simulink model "walker"  (R2021a)
settings: Solver=ode15s  StartTime=0.0  StopTime=total_time  RelTol=1e-3
values from neighbouring files (symbols this model uses):
  I_trunk_xx = trunk.mass/20 * (trunk.depth^2 + trunk.height^2)    [createWalkerWithFixedStanceFootModel.m]
  I_trunk_yy = trunk.mass/20 * (trunk.width^2 + trunk.height^2)    [createWalkerWithFixedStanceFootModel.m]
  I_trunk_zz = trunk.mass/20 * (trunk.depth^2 + trunk.width^2)    [createWalkerWithFixedStanceFootModel.m]
  shank_com_from_ankle = geometry.ankle_to_knee_z / 2    [setBiomechanicsParameters.m]
  shank_com_from_knee = geometry.ankle_to_knee_z / 2    [setBiomechanicsParameters.m]
  tau = inverseDynamics(model, theta_init, theta_dot_init)    [initialize.m]
  theta_dot_init = [0; 0; 0; 0; 0; 0]    [initialize.m]
  theta_init = [IC.left_ankle_angle; IC.left_knee_angle; IC.left_hip_angle; IC.right_hip_angle; IC.right_knee_angle; IC.right_ankle_angle]    [initialize.m]
  thigh_com_from_hip = geometry.knee_to_hip_z / 2    [setBiomechanicsParameters.m]
  thigh_com_from_knee = geometry.knee_to_hip_z / 2    [setBiomechanicsParameters.m]
undefined symbols (not defined in the file or in its folder): foot, geometry, ground, head, shank, thigh, trunk, X, Y, Z
libraries: sm_lib x75, nesl_utility x26, Contact_Forces_Lib x8, Parts_Lib x8
(part 1 of 3)
settings Model: Creator=reimajbi  LastModifiedBy=reimajbi

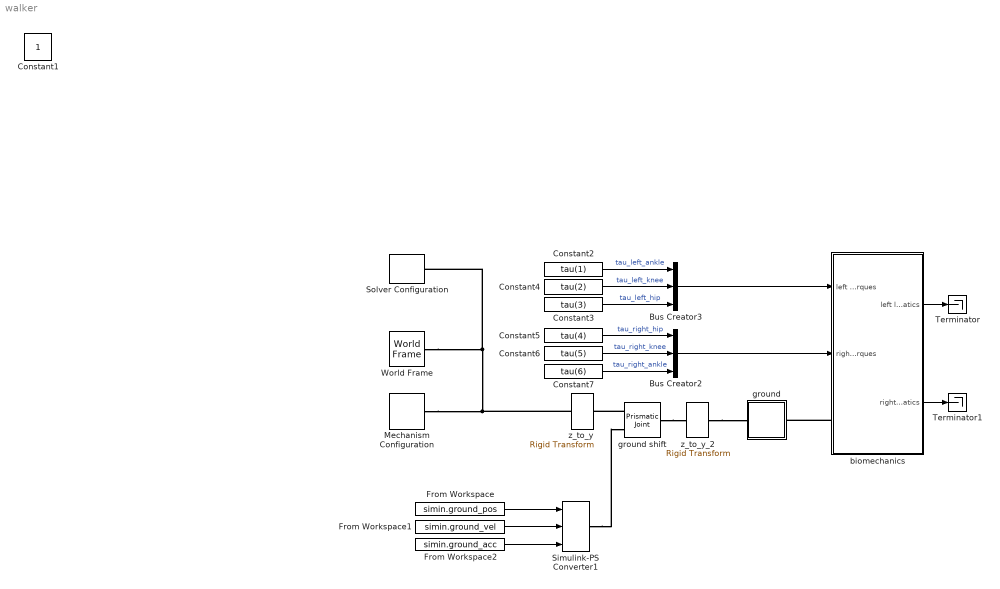
== system walker ==
  Bus Creator2 : BusCreator  Inputs=3
  Bus Creator3 : BusCreator  Inputs=3
  Constant2 : Constant  Value=tau(1)
  Constant3 : Constant  Value=tau(3)
  Constant4 : Constant  Value=tau(2)
  Constant5 : Constant  Value=tau(4)
  Constant6 : Constant  Value=tau(5)
  Constant7 : Constant  Value=tau(6)
  From Workspace : FromWorkspace  VariableName=simin.ground_pos
  From Workspace1 : FromWorkspace  VariableName=simin.ground_vel
  From Workspace2 : FromWorkspace  VariableName=simin.ground_acc
  Mechanism Configuration : sm_lib/Utilities/Mechanism Configuration  UniformGravity=Constant  GravityVector=[0 0 -9.80665]  GravityVectorUnits=m/s^2  GravityUnits=m/s^2  LinearizationDelta=0.001  JointModeTransitionNonlinearIterations=2
  Simulink-PS Converter1 : nesl_utility/Simulink-PS Converter  PhysicalDomain=network_engine_domain  SubClassName=ps_input  LeftPortType=input  RightPortType=output  PseudoPeriodic=off  Frequencies=[]  NoiseDistribution=none  NoiseParameters=[]  Unit=1  AffineConversion=off  FilteringAndDerivatives=provide  SimscapeFilterOrder=1  InputFilterTimeConstant=0.001  UdotUserProvided=2
      settings: SourceProductBaseCode=PW,SS
  Solver Configuration : nesl_utility/Solver Configuration  PhysicalDomain=network_engine_domain  SubClassName=solver  LeftPortType=input  RightPortType=generic  Tones=[]  Harmonics=[]  SimulateNoise=off  Profile=off  UseLocalSampling=off  EnableSwitchedLinearOptims=on  FrequencyDomain=off  UseCCode=off  RelTol=0.001  AbsTol=1e-06  MinStep=1e-09  ToWorkspace=off  RevertToSquareIcSolve=off  NumHomotopyIterations=100  PhasorMode=off  PhasorModeNumHarmonics=1  DoDC=off  ResidualTolerance=1e-09  UseLocalSolver=off  LocalSolverChoice=NE_BACKWARD_EULER_ADVANCER  LocalSolverSampleTime=0.001  DoFixedCost=off  MaxNonlinIter=3  MaxModeIter=2  ComputeImpulses=off  ImpulseIterations=2  LinearAlgebra=Sparse  EquationFormulation=NE_TIME_EF  DelaysMemoryBudget=1024  AutomaticFiltering=on  FilteringTimeConstant=0.001  PartitionStorageMethod=AS_NEEDED  PartitionMemoryBudget=1024  PartitionMethod=FAST
      settings: SourceProductBaseCode=PW,SS
  Terminator : Terminator
  Terminator1 : Terminator
  World Frame : sm_lib/Frames and Transforms/World Frame
  biomechanics : Subsystem
  ground : Subsystem  Tag=CustomStyle
  ground shift : sm_lib/Joints/Prismatic Joint  JointMode=Normal  SenseConstraintForce=off  SenseConstraintForceX=off  SenseConstraintForceY=off  SenseConstraintForceZ=off  SenseConstraintTorque=off  SenseConstraintTorqueX=off  SenseConstraintTorqueY=off  SenseConstraintTorqueZ=off  SenseTotalForce=off  SenseTotalForceX=off  SenseTotalForceY=off  SenseTotalForceZ=off  SenseTotalTorque=off  SenseTotalTorqueX=off  SenseTotalTorqueY=off  SenseTotalTorqueZ=off  CompositeWrenchDir=FollowerOnBase  CompositeWrenchFrame=BaseFrame  EquilibriumPosition=0  EquilibriumPositionUnits=m  SpringStiffness=0  SpringStiffnessUnits=N/m  DampingCoefficient=0  DampingCoefficientUnits=N/(m/s)  TorqueActuationMode=ComputedTorque  MotionActuationMode=InputMotion  SensePosition=off  SenseVelocity=off  SenseAcceleration=off  SenseTorqueForce=off  SenseLowerLimitTorqueForce=off  SenseUpperLimitTorqueForce=off  LowerLimitSpecify=off  LowerLimitBound=-1  LowerLimitBoundUnits=m  LowerLimitStiffness=1e6  LowerLimitStiffnessUnits=N/m  LowerLimitDamping=1e3  LowerLimitDampingUnits=N/(m/s)  LowerLimitTransitionRegionWidth=1e-4  LowerLimitTransitionRegionWidthUnits=m  UpperLimitSpecify=off  UpperLimitBound=1  UpperLimitBoundUnits=m  UpperLimitStiffness=1e6  UpperLimitStiffnessUnits=N/m  UpperLimitDamping=1e3  UpperLimitDampingUnits=N/(m/s)  UpperLimitTransitionRegionWidth=1e-4  UpperLimitTransitionRegionWidthUnits=m  PositionTargetSpecify=off  PositionTargetPriority=High  PositionTargetValue=0  PositionTargetValueUnits=m  VelocityTargetSpecify=off  VelocityTargetPriority=High  VelocityTargetValue=0  VelocityTargetValueUnits=m/s
  z_to_y : sm_lib/Frames and Transforms/Rigid Transform  TranslationMethod=None  TranslationStandardOffset=0  TranslationLengthUnit=m  TranslationStandardAxis=+Z  TranslationCartesianOffset=[0 0 0]  TranslationROffset=0  TranslationROffsetUnits=m  TranslationZOffset=0  TranslationZOffsetUnits=m  TranslationThetaOffset=0  TranslationThetaOffsetUnits=deg  RotationMethod=AlignedAxes  RotationAngleUnits=deg  RotationStandardAxis=+Z  RotationAngle=0.0  RotationArbitraryAxis=[0 0 1]  FollAlignAxisA=+Z  BaseAlignAxisA=+Y  FollAlignAxisB=+X  BaseAlignAxisB=+X  RotationSequenceAxes=FollowerAxes  RotationSequence=XYX  RotationSequenceAngles=[0 0 0]  RotationSequenceAnglesUnits=deg  RotationMatrix=[1 0 0; 0 1 0; 0 0 1]
  z_to_y_2 : sm_lib/Frames and Transforms/Rigid Transform  TranslationMethod=None  TranslationStandardOffset=0  TranslationLengthUnit=m  TranslationStandardAxis=+Z  TranslationCartesianOffset=[0 0 0]  TranslationROffset=0  TranslationROffsetUnits=m  TranslationZOffset=0  TranslationZOffsetUnits=m  TranslationThetaOffset=0  TranslationThetaOffsetUnits=deg  RotationMethod=AlignedAxes  RotationAngleUnits=deg  RotationStandardAxis=+Z  RotationAngle=0.0  RotationArbitraryAxis=[0 0 1]  FollAlignAxisA=+Z  BaseAlignAxisA=+Y  FollAlignAxisB=+X  BaseAlignAxisB=+X  RotationSequenceAxes=FollowerAxes  RotationSequence=XYX  RotationSequenceAngles=[0 0 0]  RotationSequenceAnglesUnits=deg  RotationMatrix=[1 0 0; 0 1 0; 0 0 1]
  Constant1 : Constant  IOType=siggen
  wires:
  Constant3/1 -> Bus Creator3/3  "tau_left_hip"
  Constant4/1 -> Bus Creator3/2  "tau_left_knee"
  Constant2/1 -> Bus Creator3/1  "tau_left_ankle"
  Constant5/1 -> Bus Creator2/1  "tau_right_hip"
  Constant6/1 -> Bus Creator2/2  "tau_right_knee"
  Constant7/1 -> Bus Creator2/3  "tau_right_ankle"
  Bus Creator3/1 -> biomechanics/1(left leg torques)
  Bus Creator2/1 -> biomechanics/2(right leg torques)
  biomechanics/1(left leg kinematics) -> Terminator/1
  biomechanics/2(right leg kinematics) -> Terminator1/1
  From Workspace/1 -> Simulink-PS Converter1/1
  From Workspace1/1 -> Simulink-PS Converter1/2
  From Workspace2/1 -> Simulink-PS Converter1/3
  connections:
  World Frame/RConn1 -- Mechanism Configuration/RConn1 -- z_to_y/LConn1 -- Solver Configuration/RConn1
  ground shift/LConn1 -- z_to_y/RConn1
  ground shift/RConn1 -- z_to_y_2/RConn1
  Simulink-PS Converter1/RConn1 -- ground shift/LConn2
  biomechanics/LConn1 -- ground/RConn1
  z_to_y_2/LConn1 -- ground/LConn1
